simulink library "Kitchen_Lib"  (R2023a)
settings: Solver=VariableStepAuto  StartTime=0.0  StopTime=10.0  RelTol=1e-3  EnableMultiTasking=on
undefined symbols (not defined in the file): Kitc_BusTyp_P, Kitc_BusTypSkyr_C, Kitc_ColrLedColrls_C, Kitc_ColrLedGrn_C, Kitc_ColrLedRed_C, Kitc_ColrLedYlw_C, Kitc_StDgnWtrTank_C, Kitc_StElecPlugScktOffByClmp50_P, Kitc_StsDlyBlink_C, Kitc_StsErrBlink_C, Kitc_StsFctAcvn_P, Kitc_StsInfoBlink_C, Kitc_StsKitchnOffAutoIgOff_P, Kitc_StsKitchnOffBySwt_P, Kitc_StsKitchnOffDoorLockd_P, Kitc_StsKitchnOffIgOff_P, Kitc_StsKitchnOffUv_P, Kitc_StsKitchnOnBySwt_P, Kitc_StsKitchnOnNVM_P, Kitc_StsLedOff_C, Kitc_StsLedOn_C, Kitc_StsLrgCnsAcv_P, Kitc_StTrfrAnSwtInstd_P, Kitc_StTrfrSwtInstd_P, Kitc_TiKitcRefgtrOffDly_P, Kitc_ULowrThdBat_C, Kitc_UUpprThdBat_C, Kitc_ValFalse_C, Kitc_ValPwmFreq2_C, Kitc_ValPwmFreq_C, Kitc_ValTrue_C
libraries: MAN_Library x50, E2E_Lib x3
(part 4 of 13)

== system Kitchen_Lib/Kitchen/100ms/Kitchn/Subsystem1/Subsystem19/Trfr ==
  note: Kitc_StTrfrHiSide
  note: Kitc_StTrfrLoSide signal is deleted.
  "GW_StClmp50Off3Sec " : Inport
  "GW_StUvNormPrio " : Inport  Port=2
  ABat_StAddlBatInstd : Inport  Port=3
  GW_StEngRung : Inport  Port=4
  GW_StClmp15 : Inport  Port=5
  Kitc_StsKitcAcv : Inport  Port=6
  "GW_StStrtNew " : Inport  Port=7
  "Kitc_StTrfrSwt " : Inport  Port=8
  Kitc_StTrfrSwtUpprPart : Inport  Port=9
  Kitc_StTrfrSwtTopBtn : Inport  Port=10
  Kitc_StTrfrBotmBtm : Inport  Port=11
  Kitc_StTrfrWoutNewStrt : Inport  Port=12
  001_AutomaticControlKitchenRelease : Subsystem
  002_FlipFlop : Subsystem
  Constant : Constant  Value=Kitc_StTrfrSwtInstd_P
  Constant1 : Constant  Value=Kitc_StTrfrAnSwtInstd_P
  "Constant1                                                                 " : Subsystem  AncestorBlock=MAN_Library/TimeConstant  mask{hours=0, minutes=0, seconds=0, miliseconds=50}
      mask prompts: hours "Hour"
      mask DialogControl TimeConstant Prompt: Time Constant
      mask Display:
      | timeDraw = 'Time#';
      | if( hours == 0 && minutes == 0 && seconds == 0 && miliseconds == 0)
      |     timeDraw = strcat(timeDraw,'0secs'),
      | else
      |     if( hours ~= 0)
      |         timeDraw = strcat(timeDraw,num2str(hours),'hours');
      |     end
      |     if( minutes ~= 0)
      |         timeDraw = strcat(timeDraw,num2str(minutes),'min');
      |     end
      |     if( seconds ~= 0)
      |         timeDraw = strcat(timeDraw,num2str(seconds),'sec');
      |     end
      |     if( miliseconds ~= 0)
      |         timeDraw = strcat(timeDraw,num2str(miliseconds),'ms');
      |     end
      | end
      | fprintf(timeDraw);
  Constant2 : Constant  Value=Kitc_ValTrue_C
  Data Store Read : DataStoreRead  DataStoreName=Kitc_StTrfrSwtInstdNv  IndexOptions=Index vector (dialog)  Indices=1  OutputSizes=1
  Data Store Read1 : DataStoreRead  DataStoreName=Kitc_StTrfrAnSwtInstdNv  IndexOptions=Index vector (dialog)  Indices=1  OutputSizes=1
  Data Type Conversion : DataTypeConversion  OutDataTypeStr=boolean  SaturateOnIntegerOverflow=off  RndMeth=Floor
  Data Type Conversion1 : DataTypeConversion  OutDataTypeStr=boolean  SaturateOnIntegerOverflow=off  RndMeth=Floor
  Logical Operator : Logic  Operator=NOT  AllPortsSameDT=off  OutDataTypeStr=boolean
  Logical Operator1 : Logic  Operator=OR  Inputs=3  AllPortsSameDT=off  OutDataTypeStr=boolean
  Logical Operator2 : Logic  AllPortsSameDT=off  OutDataTypeStr=boolean
  Logical Operator5 : Logic  Operator=NOT  AllPortsSameDT=off  OutDataTypeStr=boolean
  Multiport Switch : MultiPortSwitch  DataPortOrder=Zero-based contiguous  Inputs=2  zeroidx=on  SaturateOnIntegerOverflow=off  InputSameDT=off
  Switch : Switch  Criteria=u2 ~= 0  SaturateOnIntegerOverflow=off  InputSameDT=off
  Switch1 : Switch  Criteria=u2 ~= 0  SaturateOnIntegerOverflow=off  InputSameDT=off
  Terminator : Terminator
  TurnOnDelay : Subsystem  AncestorBlock=MAN_Library/TurnOnDelay  mask(Turn On Delay){CycleTime=Cycle Time: 10 Ms}
      mask prompts: CycleTime "Select the Cycle Time:"
      mask help:
      | This is an EDGE DELAY where the turning-on edge is delayed. The delay period is entered at input PT. Output Q is set on TRUE after turning on input IN, only after the delay period is over. Output ET counts the time - beginning with the occurrence of the positive edge - until the value set at PT has been reached. The output ET shows the expired time since turning input IN on until the input state of IN is put through to output Q.
      |
      | IN : Timer starting bit
      | PT : Preset time of timer
      | Q  : Time up flag
      | ET : Current value of timer
      mask TypeOptions CycleTime: Cycle Time: 1 Ms | Cycle Time: 10 Ms | Cycle Time: 100 Ms | Cycle Time: 1000 Ms
      mask Display:
      | disp('{\bf\fontsize{18}Turn On Delay}', 'texmode','on');
      | 
      | port_label('input', 1,'IN');
      | port_label('input', 2,'PT');
      | port_label('output',1,'Q');
      | port_label('output',2,'ET');
  Kitc_StTrfr : Outport
  Kitc_StTrfrInstd : Outport  Port=2
  wires:
  [Kitc_StTrfrSwtUpprPart] -> Logical Operator/1
  Data Type Conversion1/1 -> Switch1/2
  Data Type Conversion/1 -> Switch/2
  Switch1/1 -> Logical Operator1/3
  Constant1/1 -> Switch1/3
  Data Store Read1/1 -> Data Type Conversion1/1, Switch1/1
  Switch/1 -> Logical Operator1/2
  Data Store Read/1 -> Data Type Conversion/1, Switch/1
  Constant/1 -> Switch/3
  Kitc_StTrfrWoutNewStrt/1 -> 002_FlipFlop/11(Kitc_StTrfrWoutNewStrt)
  "GW_StStrtNew "/1 -> 002_FlipFlop/10("GW_StStrtNew ")
  Kitc_StTrfrBotmBtm/1 -> 002_FlipFlop/9(Kitc_StTrfrBotmBtm)
  Logical Operator/1 -> 002_FlipFlop/8(Kitc_StTrfrSwtLowrPart)
  Kitc_StTrfrSwtTopBtn/1 -> 002_FlipFlop/7(Kitc_StTrfrSwtTopBtn)
  Kitc_StTrfrSwtUpprPart/1 -> [Kitc_StTrfrSwtUpprPart], 002_FlipFlop/6(Kitc_StTrfrSwtUpprPart)
  GW_StClmp15/1 -> 002_FlipFlop/1(GW_StClmp15), 001_AutomaticControlKitchenRelease/5(GW_StClmp15)
  "GW_StUvNormPrio "/1 -> 002_FlipFlop/2("GW_StUvNormPrio "), 001_AutomaticControlKitchenRelease/4("GW_StUvNormPrio ")
  Kitc_StsKitcAcv/1 -> 001_AutomaticControlKitchenRelease/1(Kitc_StsKitcAcv)
  GW_StEngRung/1 -> 002_FlipFlop/3(GW_StEngRung), 001_AutomaticControlKitchenRelease/3(GW_StEngRung)
  ABat_StAddlBatInstd/1 -> 002_FlipFlop/4(ABat_StAddlBatInstd), 001_AutomaticControlKitchenRelease/2(ABat_StAddlBatInstd)
  Logical Operator1/1 -> Multiport Switch/1, 002_FlipFlop/5(TrfrSwt)
  001_AutomaticControlKitchenRelease/1(Kitchen) -> Multiport Switch/2
  Logical Operator5/1 -> Logical Operator2/1
  Constant2/1 -> Kitc_StTrfrInstd/1
  Multiport Switch/1 -> Logical Operator2/2
  "Kitc_StTrfrSwt "/1 -> Logical Operator1/1
  "Constant1                                                                 "/1(time) -> TurnOnDelay/2(TurnOnDelayThreshold)
  TurnOnDelay/1(TurnOnDelayFlag) -> Kitc_StTrfr/1
  Logical Operator2/1 -> TurnOnDelay/1(TurnOnDelayEnable)
  "GW_StClmp50Off3Sec "/1 -> Logical Operator5/1
  TurnOnDelay/2(TurnOnDelayExpiredTime) -> Terminator/1
  002_FlipFlop/1(Fnc_On) -> Multiport Switch/3

== system Kitchen_Lib/Kitchen/100ms/Kitchn/Subsystem1/Subsystem19/WaterTankEmptyDiagnostic ==
  Kitc_StsWtrTankEmpty : Inport
  "GW_StrtLock " : Inport  Port=2
  "GW_StClmp15On3Sec " : Inport  Port=3
  "Constant                                         " : Subsystem  AncestorBlock=MAN_Library/TimeConstant  mask{hours=0, minutes=0, seconds=3, miliseconds=0}
      mask prompts: hours "Hour"
      mask DialogControl TimeConstant Prompt: Time Constant
      mask Display:
      | timeDraw = 'Time#';
      | if( hours == 0 && minutes == 0 && seconds == 0 && miliseconds == 0)
      |     timeDraw = strcat(timeDraw,'0secs'),
      | else
      |     if( hours ~= 0)
      |         timeDraw = strcat(timeDraw,num2str(hours),'hours');
      |     end
      |     if( minutes ~= 0)
      |         timeDraw = strcat(timeDraw,num2str(minutes),'min');
      |     end
      |     if( seconds ~= 0)
      |         timeDraw = strcat(timeDraw,num2str(seconds),'sec');
      |     end
      |     if( miliseconds ~= 0)
      |         timeDraw = strcat(timeDraw,num2str(miliseconds),'ms');
      |     end
      | end
      | fprintf(timeDraw);
  "Constant1                                        " : Subsystem  AncestorBlock=MAN_Library/TimeConstant  mask{hours=0, minutes=0, seconds=30, miliseconds=0}
      mask prompts: hours "Hour"
      mask DialogControl TimeConstant Prompt: Time Constant
      mask Display:
      | timeDraw = 'Time#';
      | if( hours == 0 && minutes == 0 && seconds == 0 && miliseconds == 0)
      |     timeDraw = strcat(timeDraw,'0secs'),
      | else
      |     if( hours ~= 0)
      |         timeDraw = strcat(timeDraw,num2str(hours),'hours');
      |     end
      |     if( minutes ~= 0)
      |         timeDraw = strcat(timeDraw,num2str(minutes),'min');
      |     end
      |     if( seconds ~= 0)
      |         timeDraw = strcat(timeDraw,num2str(seconds),'sec');
      |     end
      |     if( miliseconds ~= 0)
      |         timeDraw = strcat(timeDraw,num2str(miliseconds),'ms');
      |     end
      | end
      | fprintf(timeDraw);
  "Constant2                                        " : Subsystem  AncestorBlock=MAN_Library/TimeConstant  mask{hours=0, minutes=1, seconds=0, miliseconds=0}
      mask prompts: hours "Hour"
      mask DialogControl TimeConstant Prompt: Time Constant
      mask Display:
      | timeDraw = 'Time#';
      | if( hours == 0 && minutes == 0 && seconds == 0 && miliseconds == 0)
      |     timeDraw = strcat(timeDraw,'0secs'),
      | else
      |     if( hours ~= 0)
      |         timeDraw = strcat(timeDraw,num2str(hours),'hours');
      |     end
      |     if( minutes ~= 0)
      |         timeDraw = strcat(timeDraw,num2str(minutes),'min');
      |     end
      |     if( seconds ~= 0)
      |         timeDraw = strcat(timeDraw,num2str(seconds),'sec');
      |     end
      |     if( miliseconds ~= 0)
      |         timeDraw = strcat(timeDraw,num2str(miliseconds),'ms');
      |     end
      | end
      | fprintf(timeDraw);
  Constant8 : Constant  Value=Kitc_ValTrue_C
  DIAG : Subsystem
  Diagno sticsDebouncing : Subsystem  AncestorBlock=MAN_Library/DiagnosticsDebouncing  mask(Diagnostics Debouncing){CycleTime=Cycle Time: 10 Ms}
      mask prompts: CycleTime "Select the Cycle Time:"
      mask TypeOptions CycleTime: Cycle Time: 1 Ms | Cycle Time: 10 Ms | Cycle Time: 100 Ms | Cycle Time: 1000 Ms
      mask Display:
      | %fprintf('PulseGenerator');
      | 
      | port_label('input', 1,'Error');
      | port_label('input', 2,'StartLock');
      | port_label('input', 3,'IgnitionStatus');
      | port_label('input', 4,'OnDelay');
      | port_label('input', 5,'OffDelay');
      | port_label('output',1,'DiagnosticFlag');
  Terminator : Terminator
  TurnOffDelay : Subsystem  AncestorBlock=MAN_Library/TurnOffDelay  mask(Turn Off Delay){CycleTime=Cycle Time: 10 Ms}
      mask prompts: CycleTime "Select the Cycle Time:"
      mask help:
      | This is an EDGE DELAY where the turning-off edge is delayed. The delay period is entered at input PT. The output Q is reset after turning off input IN, only after the delay period is over. Output ET counts the time - beginning with the occurrence of the negative edge - until the value set at PT has been reached. The output ET shows the expired time since turning input IN off until the input state of IN is put through to output Q.
      |
      | IN : Timer starting bit
      | PT : Preset time of timer
      | Q  : Time pulse flag
      | ET : Current value of timer
      mask TypeOptions CycleTime: Cycle Time: 1 Ms | Cycle Time: 10 Ms | Cycle Time: 100 Ms | Cycle Time: 1000 Ms
      mask Display:
      | disp('{\bf\fontsize{18}Turn Off Delay}', 'texmode','on');
      | 
      | port_label('input', 1,'IN');
      | port_label('input', 2,'PT');
      | port_label('output',1,'Q');
      | port_label('output',2,'ET');
  Kitc_EidWtrTankEmpty : Outport
  Kitch_dispWtrTnkLvlWrng : Outport  Port=2
  wires:
  "GW_StrtLock "/1 -> Diagno sticsDebouncing/2(StartLock)
  "GW_StClmp15On3Sec "/1 -> Diagno sticsDebouncing/3(IgnitionStatus)
  TurnOffDelay/1(TurnOffDelayFlag) -> Diagno sticsDebouncing/1(Error), Kitch_dispWtrTnkLvlWrng/1
  "Constant                                         "/1(time) -> TurnOffDelay/2(TurnOffDelayThreshold)
  "Constant1                                        "/1(time) -> Diagno sticsDebouncing/4(OnDelay)
  "Constant2                                        "/1(time) -> Diagno sticsDebouncing/5(OffDelay)
  Kitc_StsWtrTankEmpty/1 -> TurnOffDelay/1(TurnOffDelayEnable)
  TurnOffDelay/2(TurnOffDelayExpiredTime) -> Terminator/1
  Diagno sticsDebouncing/1(DiagnosticFlag) -> Kitc_EidWtrTankEmpty/1, DIAG/1(In1)
  Constant8/1 -> DIAG/2(In2)

== system Kitchen_Lib/Kitchen/100ms/Kitchn/Subsystem1/Subsystem2/BOOLEAN_TO_UINT8_Signals ==
  BOOLEAN_TO_UINT8_SignalIn : Inport
  Constant : Constant  Value=uint8(0)
  Constant1 : Constant  Value=uint8(1)
  Constant2 : Constant  Value=uint8(2)
  Constant3 : Constant  Value=uint8(3)
  Data Type Conversion : DataTypeConversion  OutDataTypeStr=uint8  SaturateOnIntegerOverflow=off  RndMeth=Floor
  Relational Operator{,1..3} (4 alike) : RelationalOperator  Operator===  OutDataTypeStr=boolean  InputSameDT=off
  SignalOff : Outport
  Signal|On : Outport  Port=2
  Error : Outport  Port=3
  NotInstalled_NotAvailable : Outport  Port=4
  wires:
  Relational Operator3/1 -> NotInstalled_NotAvailable/1
  Relational Operator2/1 -> Error/1
  Relational Operator1/1 -> Signal|On/1
  Relational Operator/1 -> SignalOff/1
  Data Type Conversion/1 -> Relational Operator/1, Relational Operator2/1, Relational Operator3/1, Relational Operator1/1
  Constant2/1 -> Relational Operator2/2
  Constant/1 -> Relational Operator/2
  BOOLEAN_TO_UINT8_SignalIn/1 -> Data Type Conversion/1
  Constant3/1 -> Relational Operator3/2
  Constant1/1 -> Relational Operator1/2

== system Kitchen_Lib/Kitchen/100ms/Kitchn/Subsystem1/Subsystem20/UINT32_Signal ==
  UINT32_SignalIn : Inport
  Constant : Constant  Value=uint32(0)
  Constant1 : Constant  Value=uint32(1)
  Constant2 : Constant  Value=uint32(4294967294)
  Constant3 : Constant  Value=uint32(4294967295)
  Data Type Conversion : DataTypeConversion  OutDataTypeStr=uint32  SaturateOnIntegerOverflow=off  RndMeth=Floor
  Relational Operator{,1..3} (4 alike) : RelationalOperator  Operator===  OutDataTypeStr=boolean  InputSameDT=off
  Terminator : Terminator
  Terminator1 : Terminator
  Error : Outport
  NotInstalled_NotAvailable : Outport  Port=2
  wires:
  Relational Operator3/1 -> NotInstalled_NotAvailable/1
  Relational Operator2/1 -> Error/1
  Data Type Conversion/1 -> Relational Operator/1, Relational Operator1/1, Relational Operator2/1, Relational Operator3/1
  Constant/1 -> Relational Operator/2
  UINT32_SignalIn/1 -> Data Type Conversion/1
  Constant3/1 -> Relational Operator3/2
  Constant1/1 -> Relational Operator1/2
  Relational Operator/1 -> Terminator/1
  Relational Operator1/1 -> Terminator1/1
  Constant2/1 -> Relational Operator2/2

== system Kitchen_Lib/Kitchen/100ms/Kitchn/Subsystem1/Subsystem21/SignalE2EStandardBool ==
  Sıgnal_In : Inport
  Error_In : Inport  Port=2
  NotAvailable : Inport  Port=3
  Constant10 : Constant  Value=uint8(2)
  Constant12 : Constant  Value=uint8(3)
  Constant7 : Constant  Value=uint8(1)
  Constant9 : Constant  Value=uint8(0)
  Data Type Conversion1 : DataTypeConversion  OutDataTypeStr=boolean  SaturateOnIntegerOverflow=off  RndMeth=Floor
  Data Type Conversion2 : DataTypeConversion  OutDataTypeStr=boolean  SaturateOnIntegerOverflow=off  RndMeth=Floor
  Data Type Conversion3 : DataTypeConversion  OutDataTypeStr=boolean  SaturateOnIntegerOverflow=off  RndMeth=Floor
  Multiport Switch : MultiPortSwitch  DataPortOrder=Zero-based contiguous  Inputs=2  zeroidx=on  SaturateOnIntegerOverflow=off  InputSameDT=off
  Multiport Switch1 : MultiPortSwitch  DataPortOrder=Zero-based contiguous  Inputs=2  zeroidx=on  SaturateOnIntegerOverflow=off  InputSameDT=off
  Multiport Switch2 : MultiPortSwitch  DataPortOrder=Zero-based contiguous  Inputs=2  zeroidx=on  SaturateOnIntegerOverflow=off  InputSameDT=off
  Signal_Out : Outport
  wires:
  Multiport Switch2/1 -> Signal_Out/1
  Data Type Conversion3/1 -> Multiport Switch2/1
  Data Type Conversion2/1 -> Multiport Switch1/1
  Constant12/1 -> Multiport Switch2/3
  NotAvailable/1 -> Data Type Conversion3/1
  Multiport Switch1/1 -> Multiport Switch2/2
  Error_In/1 -> Data Type Conversion2/1
  Multiport Switch/1 -> Multiport Switch1/2
  Constant10/1 -> Multiport Switch1/3
  Constant9/1 -> Multiport Switch/2
  Constant7/1 -> Multiport Switch/3
  Data Type Conversion1/1 -> Multiport Switch/1
  Sıgnal_In/1 -> Data Type Conversion1/1

== system Kitchen_Lib/Kitchen/100ms/Kitchn/Subsystem1/Subsystem22/SignalE2EStandardU16 ==
  Sıgnal_In : Inport
  Error_In : Inport  Port=2
  NotAvailable : Inport  Port=3
  Constant10 : Constant  Value=uint16(65534)
  Constant12 : Constant  Value=uint16(65535)
  Constant9 : Constant  Value=uint16(0)
  Data Type Conversion1 : DataTypeConversion  OutDataTypeStr=boolean  SaturateOnIntegerOverflow=off  RndMeth=Floor
  Data Type Conversion2 : DataTypeConversion  OutDataTypeStr=boolean  SaturateOnIntegerOverflow=off  RndMeth=Floor
  Data Type Conversion3 : DataTypeConversion  OutDataTypeStr=boolean  SaturateOnIntegerOverflow=off  RndMeth=Floor
  Multiport Switch : MultiPortSwitch  DataPortOrder=Zero-based contiguous  Inputs=2  zeroidx=on  SaturateOnIntegerOverflow=off  InputSameDT=off
  Multiport Switch1 : MultiPortSwitch  DataPortOrder=Zero-based contiguous  Inputs=2  zeroidx=on  SaturateOnIntegerOverflow=off  InputSameDT=off
  Multiport Switch2 : MultiPortSwitch  DataPortOrder=Zero-based contiguous  Inputs=2  zeroidx=on  SaturateOnIntegerOverflow=off  InputSameDT=off
  Signal_Out : Outport
  wires:
  Data Type Conversion1/1 -> Multiport Switch/1
  Sıgnal_In/1 -> Data Type Conversion1/1, Multiport Switch/3
  Constant9/1 -> Multiport Switch/2
  Constant10/1 -> Multiport Switch1/3
  Multiport Switch/1 -> Multiport Switch1/2
  Error_In/1 -> Data Type Conversion2/1
  Multiport Switch1/1 -> Multiport Switch2/2
  NotAvailable/1 -> Data Type Conversion3/1
  Constant12/1 -> Multiport Switch2/3
  Data Type Conversion2/1 -> Multiport Switch1/1
  Data Type Conversion3/1 -> Multiport Switch2/1
  Multiport Switch2/1 -> Signal_Out/1

== system Kitchen_Lib/Kitchen/100ms/Kitchn/Subsystem1/Subsystem23/SignalE2EStandardU16 ==
  Sıgnal_In : Inport
  Error_In : Inport  Port=2
  NotAvailable : Inport  Port=3
  Constant10 : Constant  Value=uint16(65534)
  Constant12 : Constant  Value=uint16(65535)
  Constant9 : Constant  Value=uint16(0)
  Data Type Conversion1 : DataTypeConversion  OutDataTypeStr=boolean  SaturateOnIntegerOverflow=off  RndMeth=Floor
  Data Type Conversion2 : DataTypeConversion  OutDataTypeStr=boolean  SaturateOnIntegerOverflow=off  RndMeth=Floor
  Data Type Conversion3 : DataTypeConversion  OutDataTypeStr=boolean  SaturateOnIntegerOverflow=off  RndMeth=Floor
  Multiport Switch : MultiPortSwitch  DataPortOrder=Zero-based contiguous  Inputs=2  zeroidx=on  SaturateOnIntegerOverflow=off  InputSameDT=off
  Multiport Switch1 : MultiPortSwitch  DataPortOrder=Zero-based contiguous  Inputs=2  zeroidx=on  SaturateOnIntegerOverflow=off  InputSameDT=off
  Multiport Switch2 : MultiPortSwitch  DataPortOrder=Zero-based contiguous  Inputs=2  zeroidx=on  SaturateOnIntegerOverflow=off  InputSameDT=off
  Signal_Out : Outport
  wires:
  Data Type Conversion1/1 -> Multiport Switch/1
  Sıgnal_In/1 -> Data Type Conversion1/1, Multiport Switch/3
  Constant9/1 -> Multiport Switch/2
  Constant10/1 -> Multiport Switch1/3
  Multiport Switch/1 -> Multiport Switch1/2
  Error_In/1 -> Data Type Conversion2/1
  Multiport Switch1/1 -> Multiport Switch2/2
  NotAvailable/1 -> Data Type Conversion3/1
  Constant12/1 -> Multiport Switch2/3
  Data Type Conversion2/1 -> Multiport Switch1/1
  Data Type Conversion3/1 -> Multiport Switch2/1
  Multiport Switch2/1 -> Signal_Out/1

== system Kitchen_Lib/Kitchen/100ms/Kitchn/Subsystem1/Subsystem24/SignalE2EStandardBool ==
  Sıgnal_In : Inport
  Error_In : Inport  Port=2
  NotAvailable : Inport  Port=3
  Constant10 : Constant  Value=uint8(2)
  Constant12 : Constant  Value=uint8(3)
  Constant7 : Constant  Value=uint8(1)
  Constant9 : Constant  Value=uint8(0)
  Data Type Conversion1 : DataTypeConversion  OutDataTypeStr=boolean  SaturateOnIntegerOverflow=off  RndMeth=Floor
  Data Type Conversion2 : DataTypeConversion  OutDataTypeStr=boolean  SaturateOnIntegerOverflow=off  RndMeth=Floor
  Data Type Conversion3 : DataTypeConversion  OutDataTypeStr=boolean  SaturateOnIntegerOverflow=off  RndMeth=Floor
  Multiport Switch : MultiPortSwitch  DataPortOrder=Zero-based contiguous  Inputs=2  zeroidx=on  SaturateOnIntegerOverflow=off  InputSameDT=off
  Multiport Switch1 : MultiPortSwitch  DataPortOrder=Zero-based contiguous  Inputs=2  zeroidx=on  SaturateOnIntegerOverflow=off  InputSameDT=off
  Multiport Switch2 : MultiPortSwitch  DataPortOrder=Zero-based contiguous  Inputs=2  zeroidx=on  SaturateOnIntegerOverflow=off  InputSameDT=off
  Signal_Out : Outport
  wires:
  Multiport Switch2/1 -> Signal_Out/1
  Data Type Conversion3/1 -> Multiport Switch2/1
  Data Type Conversion2/1 -> Multiport Switch1/1
  Constant12/1 -> Multiport Switch2/3
  NotAvailable/1 -> Data Type Conversion3/1
  Multiport Switch1/1 -> Multiport Switch2/2
  Error_In/1 -> Data Type Conversion2/1
  Multiport Switch/1 -> Multiport Switch1/2
  Constant10/1 -> Multiport Switch1/3
  Constant9/1 -> Multiport Switch/2
  Constant7/1 -> Multiport Switch/3
  Data Type Conversion1/1 -> Multiport Switch/1
  Sıgnal_In/1 -> Data Type Conversion1/1

== system Kitchen_Lib/Kitchen/100ms/Kitchn/Subsystem1/Subsystem25/SignalE2EStandardBool ==
  Sıgnal_In : Inport
  Error_In : Inport  Port=2
  NotAvailable : Inport  Port=3
  Constant10 : Constant  Value=uint8(2)
  Constant12 : Constant  Value=uint8(3)
  Constant7 : Constant  Value=uint8(1)
  Constant9 : Constant  Value=uint8(0)
  Data Type Conversion1 : DataTypeConversion  OutDataTypeStr=boolean  SaturateOnIntegerOverflow=off  RndMeth=Floor
  Data Type Conversion2 : DataTypeConversion  OutDataTypeStr=boolean  SaturateOnIntegerOverflow=off  RndMeth=Floor
  Data Type Conversion3 : DataTypeConversion  OutDataTypeStr=boolean  SaturateOnIntegerOverflow=off  RndMeth=Floor
  Multiport Switch : MultiPortSwitch  DataPortOrder=Zero-based contiguous  Inputs=2  zeroidx=on  SaturateOnIntegerOverflow=off  InputSameDT=off
  Multiport Switch1 : MultiPortSwitch  DataPortOrder=Zero-based contiguous  Inputs=2  zeroidx=on  SaturateOnIntegerOverflow=off  InputSameDT=off
  Multiport Switch2 : MultiPortSwitch  DataPortOrder=Zero-based contiguous  Inputs=2  zeroidx=on  SaturateOnIntegerOverflow=off  InputSameDT=off
  Signal_Out : Outport
  wires:
  Multiport Switch2/1 -> Signal_Out/1
  Data Type Conversion3/1 -> Multiport Switch2/1
  Data Type Conversion2/1 -> Multiport Switch1/1
  Constant12/1 -> Multiport Switch2/3
  NotAvailable/1 -> Data Type Conversion3/1
  Multiport Switch1/1 -> Multiport Switch2/2
  Error_In/1 -> Data Type Conversion2/1
  Multiport Switch/1 -> Multiport Switch1/2
  Constant10/1 -> Multiport Switch1/3
  Constant9/1 -> Multiport Switch/2
  Constant7/1 -> Multiport Switch/3
  Data Type Conversion1/1 -> Multiport Switch/1
  Sıgnal_In/1 -> Data Type Conversion1/1

== system Kitchen_Lib/Kitchen/100ms/Kitchn/Subsystem1/Subsystem26/SignalE2EStandardBool ==
  Sıgnal_In : Inport
  Error_In : Inport  Port=2
  NotAvailable : Inport  Port=3
  Constant10 : Constant  Value=uint8(2)
  Constant12 : Constant  Value=uint8(3)
  Constant7 : Constant  Value=uint8(1)
  Constant9 : Constant  Value=uint8(0)
  Data Type Conversion1 : DataTypeConversion  OutDataTypeStr=boolean  SaturateOnIntegerOverflow=off  RndMeth=Floor
  Data Type Conversion2 : DataTypeConversion  OutDataTypeStr=boolean  SaturateOnIntegerOverflow=off  RndMeth=Floor
  Data Type Conversion3 : DataTypeConversion  OutDataTypeStr=boolean  SaturateOnIntegerOverflow=off  RndMeth=Floor
  Multiport Switch : MultiPortSwitch  DataPortOrder=Zero-based contiguous  Inputs=2  zeroidx=on  SaturateOnIntegerOverflow=off  InputSameDT=off
  Multiport Switch1 : MultiPortSwitch  DataPortOrder=Zero-based contiguous  Inputs=2  zeroidx=on  SaturateOnIntegerOverflow=off  InputSameDT=off
  Multiport Switch2 : MultiPortSwitch  DataPortOrder=Zero-based contiguous  Inputs=2  zeroidx=on  SaturateOnIntegerOverflow=off  InputSameDT=off
  Signal_Out : Outport
  wires:
  Multiport Switch2/1 -> Signal_Out/1
  Data Type Conversion3/1 -> Multiport Switch2/1
  Data Type Conversion2/1 -> Multiport Switch1/1
  Constant12/1 -> Multiport Switch2/3
  NotAvailable/1 -> Data Type Conversion3/1
  Multiport Switch1/1 -> Multiport Switch2/2
  Error_In/1 -> Data Type Conversion2/1
  Multiport Switch/1 -> Multiport Switch1/2
  Constant10/1 -> Multiport Switch1/3
  Constant9/1 -> Multiport Switch/2
  Constant7/1 -> Multiport Switch/3
  Data Type Conversion1/1 -> Multiport Switch/1
  Sıgnal_In/1 -> Data Type Conversion1/1

== system Kitchen_Lib/Kitchen/100ms/Kitchn/Subsystem1/Subsystem27/SignalE2EStandardBool ==
  Sıgnal_In : Inport
  Error_In : Inport  Port=2
  NotAvailable : Inport  Port=3
  Constant10 : Constant  Value=uint8(2)
  Constant12 : Constant  Value=uint8(3)
  Constant7 : Constant  Value=uint8(1)
  Constant9 : Constant  Value=uint8(0)
  Data Type Conversion1 : DataTypeConversion  OutDataTypeStr=boolean  SaturateOnIntegerOverflow=off  RndMeth=Floor
  Data Type Conversion2 : DataTypeConversion  OutDataTypeStr=boolean  SaturateOnIntegerOverflow=off  RndMeth=Floor
  Data Type Conversion3 : DataTypeConversion  OutDataTypeStr=boolean  SaturateOnIntegerOverflow=off  RndMeth=Floor
  Multiport Switch : MultiPortSwitch  DataPortOrder=Zero-based contiguous  Inputs=2  zeroidx=on  SaturateOnIntegerOverflow=off  InputSameDT=off
  Multiport Switch1 : MultiPortSwitch  DataPortOrder=Zero-based contiguous  Inputs=2  zeroidx=on  SaturateOnIntegerOverflow=off  InputSameDT=off
  Multiport Switch2 : MultiPortSwitch  DataPortOrder=Zero-based contiguous  Inputs=2  zeroidx=on  SaturateOnIntegerOverflow=off  InputSameDT=off
  Signal_Out : Outport
  wires:
  Multiport Switch2/1 -> Signal_Out/1
  Data Type Conversion3/1 -> Multiport Switch2/1
  Data Type Conversion2/1 -> Multiport Switch1/1
  Constant12/1 -> Multiport Switch2/3
  NotAvailable/1 -> Data Type Conversion3/1
  Multiport Switch1/1 -> Multiport Switch2/2
  Error_In/1 -> Data Type Conversion2/1
  Multiport Switch/1 -> Multiport Switch1/2
  Constant10/1 -> Multiport Switch1/3
  Constant9/1 -> Multiport Switch/2
  Constant7/1 -> Multiport Switch/3
  Data Type Conversion1/1 -> Multiport Switch/1
  Sıgnal_In/1 -> Data Type Conversion1/1

== system Kitchen_Lib/Kitchen/100ms/Kitchn/Subsystem1/Subsystem28/SignalE2EStandardBool ==
  Sıgnal_In : Inport
  Error_In : Inport  Port=2
  NotAvailable : Inport  Port=3
  Constant10 : Constant  Value=uint8(2)
  Constant12 : Constant  Value=uint8(3)
  Constant7 : Constant  Value=uint8(1)
  Constant9 : Constant  Value=uint8(0)
  Data Type Conversion1 : DataTypeConversion  OutDataTypeStr=boolean  SaturateOnIntegerOverflow=off  RndMeth=Floor
  Data Type Conversion2 : DataTypeConversion  OutDataTypeStr=boolean  SaturateOnIntegerOverflow=off  RndMeth=Floor
  Data Type Conversion3 : DataTypeConversion  OutDataTypeStr=boolean  SaturateOnIntegerOverflow=off  RndMeth=Floor
  Multiport Switch : MultiPortSwitch  DataPortOrder=Zero-based contiguous  Inputs=2  zeroidx=on  SaturateOnIntegerOverflow=off  InputSameDT=off
  Multiport Switch1 : MultiPortSwitch  DataPortOrder=Zero-based contiguous  Inputs=2  zeroidx=on  SaturateOnIntegerOverflow=off  InputSameDT=off
  Multiport Switch2 : MultiPortSwitch  DataPortOrder=Zero-based contiguous  Inputs=2  zeroidx=on  SaturateOnIntegerOverflow=off  InputSameDT=off
  Signal_Out : Outport
  wires:
  Multiport Switch2/1 -> Signal_Out/1
  Data Type Conversion3/1 -> Multiport Switch2/1
  Data Type Conversion2/1 -> Multiport Switch1/1
  Constant12/1 -> Multiport Switch2/3
  NotAvailable/1 -> Data Type Conversion3/1
  Multiport Switch1/1 -> Multiport Switch2/2
  Error_In/1 -> Data Type Conversion2/1
  Multiport Switch/1 -> Multiport Switch1/2
  Constant10/1 -> Multiport Switch1/3
  Constant9/1 -> Multiport Switch/2
  Constant7/1 -> Multiport Switch/3
  Data Type Conversion1/1 -> Multiport Switch/1
  Sıgnal_In/1 -> Data Type Conversion1/1

== system Kitchen_Lib/Kitchen/100ms/Kitchn/Subsystem1/Subsystem29/SignalE2EStandardBool ==
  Sıgnal_In : Inport
  Error_In : Inport  Port=2
  NotAvailable : Inport  Port=3
  Constant10 : Constant  Value=uint8(2)
  Constant12 : Constant  Value=uint8(3)
  Constant7 : Constant  Value=uint8(1)
  Constant9 : Constant  Value=uint8(0)
  Data Type Conversion1 : DataTypeConversion  OutDataTypeStr=boolean  SaturateOnIntegerOverflow=off  RndMeth=Floor
  Data Type Conversion2 : DataTypeConversion  OutDataTypeStr=boolean  SaturateOnIntegerOverflow=off  RndMeth=Floor
  Data Type Conversion3 : DataTypeConversion  OutDataTypeStr=boolean  SaturateOnIntegerOverflow=off  RndMeth=Floor
  Multiport Switch : MultiPortSwitch  DataPortOrder=Zero-based contiguous  Inputs=2  zeroidx=on  SaturateOnIntegerOverflow=off  InputSameDT=off
  Multiport Switch1 : MultiPortSwitch  DataPortOrder=Zero-based contiguous  Inputs=2  zeroidx=on  SaturateOnIntegerOverflow=off  InputSameDT=off
  Multiport Switch2 : MultiPortSwitch  DataPortOrder=Zero-based contiguous  Inputs=2  zeroidx=on  SaturateOnIntegerOverflow=off  InputSameDT=off
  Signal_Out : Outport
  wires:
  Multiport Switch2/1 -> Signal_Out/1
  Data Type Conversion3/1 -> Multiport Switch2/1
  Data Type Conversion2/1 -> Multiport Switch1/1
  Constant12/1 -> Multiport Switch2/3
  NotAvailable/1 -> Data Type Conversion3/1
  Multiport Switch1/1 -> Multiport Switch2/2
  Error_In/1 -> Data Type Conversion2/1
  Multiport Switch/1 -> Multiport Switch1/2
  Constant10/1 -> Multiport Switch1/3
  Constant9/1 -> Multiport Switch/2
  Constant7/1 -> Multiport Switch/3
  Data Type Conversion1/1 -> Multiport Switch/1
  Sıgnal_In/1 -> Data Type Conversion1/1

== system Kitchen_Lib/Kitchen/100ms/Kitchn/Subsystem1/Subsystem3/BOOLEAN_TO_UINT8_Signals ==
  BOOLEAN_TO_UINT8_SignalIn : Inport
  Constant : Constant  Value=uint8(0)
  Constant1 : Constant  Value=uint8(1)
  Constant2 : Constant  Value=uint8(2)
  Constant3 : Constant  Value=uint8(3)
  Data Type Conversion : DataTypeConversion  OutDataTypeStr=uint8  SaturateOnIntegerOverflow=off  RndMeth=Floor
  Relational Operator{,1..3} (4 alike) : RelationalOperator  Operator===  OutDataTypeStr=boolean  InputSameDT=off
  SignalOff : Outport
  Signal|On : Outport  Port=2
  Error : Outport  Port=3
  NotInstalled_NotAvailable : Outport  Port=4
  wires:
  Relational Operator3/1 -> NotInstalled_NotAvailable/1
  Relational Operator2/1 -> Error/1
  Relational Operator1/1 -> Signal|On/1
  Relational Operator/1 -> SignalOff/1
  Data Type Conversion/1 -> Relational Operator/1, Relational Operator2/1, Relational Operator3/1, Relational Operator1/1
  Constant2/1 -> Relational Operator2/2
  Constant/1 -> Relational Operator/2
  BOOLEAN_TO_UINT8_SignalIn/1 -> Data Type Conversion/1
  Constant3/1 -> Relational Operator3/2
  Constant1/1 -> Relational Operator1/2

== system Kitchen_Lib/Kitchen/100ms/Kitchn/Subsystem1/Subsystem30/SignalE2EStandardBool ==
  Sıgnal_In : Inport
  Error_In : Inport  Port=2
  NotAvailable : Inport  Port=3
  Constant10 : Constant  Value=uint8(2)
  Constant12 : Constant  Value=uint8(3)
  Constant7 : Constant  Value=uint8(1)
  Constant9 : Constant  Value=uint8(0)
  Data Type Conversion1 : DataTypeConversion  OutDataTypeStr=boolean  SaturateOnIntegerOverflow=off  RndMeth=Floor
  Data Type Conversion2 : DataTypeConversion  OutDataTypeStr=boolean  SaturateOnIntegerOverflow=off  RndMeth=Floor
  Data Type Conversion3 : DataTypeConversion  OutDataTypeStr=boolean  SaturateOnIntegerOverflow=off  RndMeth=Floor
  Multiport Switch : MultiPortSwitch  DataPortOrder=Zero-based contiguous  Inputs=2  zeroidx=on  SaturateOnIntegerOverflow=off  InputSameDT=off
  Multiport Switch1 : MultiPortSwitch  DataPortOrder=Zero-based contiguous  Inputs=2  zeroidx=on  SaturateOnIntegerOverflow=off  InputSameDT=off
  Multiport Switch2 : MultiPortSwitch  DataPortOrder=Zero-based contiguous  Inputs=2  zeroidx=on  SaturateOnIntegerOverflow=off  InputSameDT=off
  Signal_Out : Outport
  wires:
  Multiport Switch2/1 -> Signal_Out/1
  Data Type Conversion3/1 -> Multiport Switch2/1
  Data Type Conversion2/1 -> Multiport Switch1/1
  Constant12/1 -> Multiport Switch2/3
  NotAvailable/1 -> Data Type Conversion3/1
  Multiport Switch1/1 -> Multiport Switch2/2
  Error_In/1 -> Data Type Conversion2/1
  Multiport Switch/1 -> Multiport Switch1/2
  Constant10/1 -> Multiport Switch1/3
  Constant9/1 -> Multiport Switch/2
  Constant7/1 -> Multiport Switch/3
  Data Type Conversion1/1 -> Multiport Switch/1
  Sıgnal_In/1 -> Data Type Conversion1/1

== system Kitchen_Lib/Kitchen/100ms/Kitchn/Subsystem1/Subsystem31/SignalE2EStandardBool ==
  Sıgnal_In : Inport
  Error_In : Inport  Port=2
  NotAvailable : Inport  Port=3
  Constant10 : Constant  Value=uint8(2)
  Constant12 : Constant  Value=uint8(3)
  Constant7 : Constant  Value=uint8(1)
  Constant9 : Constant  Value=uint8(0)
  Data Type Conversion1 : DataTypeConversion  OutDataTypeStr=boolean  SaturateOnIntegerOverflow=off  RndMeth=Floor
  Data Type Conversion2 : DataTypeConversion  OutDataTypeStr=boolean  SaturateOnIntegerOverflow=off  RndMeth=Floor
  Data Type Conversion3 : DataTypeConversion  OutDataTypeStr=boolean  SaturateOnIntegerOverflow=off  RndMeth=Floor
  Multiport Switch : MultiPortSwitch  DataPortOrder=Zero-based contiguous  Inputs=2  zeroidx=on  SaturateOnIntegerOverflow=off  InputSameDT=off
  Multiport Switch1 : MultiPortSwitch  DataPortOrder=Zero-based contiguous  Inputs=2  zeroidx=on  SaturateOnIntegerOverflow=off  InputSameDT=off
  Multiport Switch2 : MultiPortSwitch  DataPortOrder=Zero-based contiguous  Inputs=2  zeroidx=on  SaturateOnIntegerOverflow=off  InputSameDT=off
  Signal_Out : Outport
  wires:
  Multiport Switch2/1 -> Signal_Out/1
  Data Type Conversion3/1 -> Multiport Switch2/1
  Data Type Conversion2/1 -> Multiport Switch1/1
  Constant12/1 -> Multiport Switch2/3
  NotAvailable/1 -> Data Type Conversion3/1
  Multiport Switch1/1 -> Multiport Switch2/2
  Error_In/1 -> Data Type Conversion2/1
  Multiport Switch/1 -> Multiport Switch1/2
  Constant10/1 -> Multiport Switch1/3
  Constant9/1 -> Multiport Switch/2
  Constant7/1 -> Multiport Switch/3
  Data Type Conversion1/1 -> Multiport Switch/1
  Sıgnal_In/1 -> Data Type Conversion1/1

== system Kitchen_Lib/Kitchen/100ms/Kitchn/Subsystem1/Subsystem32/SignalE2EStandardBool ==
  Sıgnal_In : Inport
  Error_In : Inport  Port=2
  NotAvailable : Inport  Port=3
  Constant10 : Constant  Value=uint8(2)
  Constant12 : Constant  Value=uint8(3)
  Constant7 : Constant  Value=uint8(1)
  Constant9 : Constant  Value=uint8(0)
  Data Type Conversion1 : DataTypeConversion  OutDataTypeStr=boolean  SaturateOnIntegerOverflow=off  RndMeth=Floor
  Data Type Conversion2 : DataTypeConversion  OutDataTypeStr=boolean  SaturateOnIntegerOverflow=off  RndMeth=Floor
  Data Type Conversion3 : DataTypeConversion  OutDataTypeStr=boolean  SaturateOnIntegerOverflow=off  RndMeth=Floor
  Multiport Switch : MultiPortSwitch  DataPortOrder=Zero-based contiguous  Inputs=2  zeroidx=on  SaturateOnIntegerOverflow=off  InputSameDT=off
  Multiport Switch1 : MultiPortSwitch  DataPortOrder=Zero-based contiguous  Inputs=2  zeroidx=on  SaturateOnIntegerOverflow=off  InputSameDT=off
  Multiport Switch2 : MultiPortSwitch  DataPortOrder=Zero-based contiguous  Inputs=2  zeroidx=on  SaturateOnIntegerOverflow=off  InputSameDT=off
  Signal_Out : Outport
  wires:
  Multiport Switch2/1 -> Signal_Out/1
  Data Type Conversion3/1 -> Multiport Switch2/1
  Data Type Conversion2/1 -> Multiport Switch1/1
  Constant12/1 -> Multiport Switch2/3
  NotAvailable/1 -> Data Type Conversion3/1
  Multiport Switch1/1 -> Multiport Switch2/2
  Error_In/1 -> Data Type Conversion2/1
  Multiport Switch/1 -> Multiport Switch1/2
  Constant10/1 -> Multiport Switch1/3
  Constant9/1 -> Multiport Switch/2
  Constant7/1 -> Multiport Switch/3
  Data Type Conversion1/1 -> Multiport Switch/1
  Sıgnal_In/1 -> Data Type Conversion1/1

== system Kitchen_Lib/Kitchen/100ms/Kitchn/Subsystem1/Subsystem33/SignalE2EStandardU16 ==
  Sıgnal_In : Inport
  Error_In : Inport  Port=2
  NotAvailable : Inport  Port=3
  Constant10 : Constant  Value=uint16(65534)
  Constant12 : Constant  Value=uint16(65535)
  Constant9 : Constant  Value=uint16(0)
  Data Type Conversion1 : DataTypeConversion  OutDataTypeStr=boolean  SaturateOnIntegerOverflow=off  RndMeth=Floor
  Data Type Conversion2 : DataTypeConversion  OutDataTypeStr=boolean  SaturateOnIntegerOverflow=off  RndMeth=Floor
  Data Type Conversion3 : DataTypeConversion  OutDataTypeStr=boolean  SaturateOnIntegerOverflow=off  RndMeth=Floor
  Multiport Switch : MultiPortSwitch  DataPortOrder=Zero-based contiguous  Inputs=2  zeroidx=on  SaturateOnIntegerOverflow=off  InputSameDT=off
  Multiport Switch1 : MultiPortSwitch  DataPortOrder=Zero-based contiguous  Inputs=2  zeroidx=on  SaturateOnIntegerOverflow=off  InputSameDT=off
  Multiport Switch2 : MultiPortSwitch  DataPortOrder=Zero-based contiguous  Inputs=2  zeroidx=on  SaturateOnIntegerOverflow=off  InputSameDT=off
  Signal_Out : Outport
  wires:
  Data Type Conversion1/1 -> Multiport Switch/1
  Sıgnal_In/1 -> Data Type Conversion1/1, Multiport Switch/3
  Constant9/1 -> Multiport Switch/2
  Constant10/1 -> Multiport Switch1/3
  Multiport Switch/1 -> Multiport Switch1/2
  Error_In/1 -> Data Type Conversion2/1
  Multiport Switch1/1 -> Multiport Switch2/2
  NotAvailable/1 -> Data Type Conversion3/1
  Constant12/1 -> Multiport Switch2/3
  Data Type Conversion2/1 -> Multiport Switch1/1
  Data Type Conversion3/1 -> Multiport Switch2/1
  Multiport Switch2/1 -> Signal_Out/1

== system Kitchen_Lib/Kitchen/100ms/Kitchn/Subsystem1/Subsystem34/SignalE2EStandardU16 ==
  Sıgnal_In : Inport
  Error_In : Inport  Port=2
  NotAvailable : Inport  Port=3
  Constant10 : Constant  Value=uint16(65534)
  Constant12 : Constant  Value=uint16(65535)
  Constant9 : Constant  Value=uint16(0)
  Data Type Conversion1 : DataTypeConversion  OutDataTypeStr=boolean  SaturateOnIntegerOverflow=off  RndMeth=Floor
  Data Type Conversion2 : DataTypeConversion  OutDataTypeStr=boolean  SaturateOnIntegerOverflow=off  RndMeth=Floor
  Data Type Conversion3 : DataTypeConversion  OutDataTypeStr=boolean  SaturateOnIntegerOverflow=off  RndMeth=Floor
  Multiport Switch : MultiPortSwitch  DataPortOrder=Zero-based contiguous  Inputs=2  zeroidx=on  SaturateOnIntegerOverflow=off  InputSameDT=off
  Multiport Switch1 : MultiPortSwitch  DataPortOrder=Zero-based contiguous  Inputs=2  zeroidx=on  SaturateOnIntegerOverflow=off  InputSameDT=off
  Multiport Switch2 : MultiPortSwitch  DataPortOrder=Zero-based contiguous  Inputs=2  zeroidx=on  SaturateOnIntegerOverflow=off  InputSameDT=off
  Signal_Out : Outport
  wires:
  Data Type Conversion1/1 -> Multiport Switch/1
  Sıgnal_In/1 -> Data Type Conversion1/1, Multiport Switch/3
  Constant9/1 -> Multiport Switch/2
  Constant10/1 -> Multiport Switch1/3
  Multiport Switch/1 -> Multiport Switch1/2
  Error_In/1 -> Data Type Conversion2/1
  Multiport Switch1/1 -> Multiport Switch2/2
  NotAvailable/1 -> Data Type Conversion3/1
  Constant12/1 -> Multiport Switch2/3
  Data Type Conversion2/1 -> Multiport Switch1/1
  Data Type Conversion3/1 -> Multiport Switch2/1
  Multiport Switch2/1 -> Signal_Out/1

== system Kitchen_Lib/Kitchen/100ms/Kitchn/Subsystem1/Subsystem35/SignalE2EStandardU16 ==
  Sıgnal_In : Inport
  Error_In : Inport  Port=2
  NotAvailable : Inport  Port=3
  Constant10 : Constant  Value=uint16(65534)
  Constant12 : Constant  Value=uint16(65535)
  Constant9 : Constant  Value=uint16(0)
  Data Type Conversion1 : DataTypeConversion  OutDataTypeStr=boolean  SaturateOnIntegerOverflow=off  RndMeth=Floor
  Data Type Conversion2 : DataTypeConversion  OutDataTypeStr=boolean  SaturateOnIntegerOverflow=off  RndMeth=Floor
  Data Type Conversion3 : DataTypeConversion  OutDataTypeStr=boolean  SaturateOnIntegerOverflow=off  RndMeth=Floor
  Multiport Switch : MultiPortSwitch  DataPortOrder=Zero-based contiguous  Inputs=2  zeroidx=on  SaturateOnIntegerOverflow=off  InputSameDT=off
  Multiport Switch1 : MultiPortSwitch  DataPortOrder=Zero-based contiguous  Inputs=2  zeroidx=on  SaturateOnIntegerOverflow=off  InputSameDT=off
  Multiport Switch2 : MultiPortSwitch  DataPortOrder=Zero-based contiguous  Inputs=2  zeroidx=on  SaturateOnIntegerOverflow=off  InputSameDT=off
  Signal_Out : Outport
  wires:
  Data Type Conversion1/1 -> Multiport Switch/1
  Sıgnal_In/1 -> Data Type Conversion1/1, Multiport Switch/3
  Constant9/1 -> Multiport Switch/2
  Constant10/1 -> Multiport Switch1/3
  Multiport Switch/1 -> Multiport Switch1/2
  Error_In/1 -> Data Type Conversion2/1
  Multiport Switch1/1 -> Multiport Switch2/2
  NotAvailable/1 -> Data Type Conversion3/1
  Constant12/1 -> Multiport Switch2/3
  Data Type Conversion2/1 -> Multiport Switch1/1
  Data Type Conversion3/1 -> Multiport Switch2/1
  Multiport Switch2/1 -> Signal_Out/1

== system Kitchen_Lib/Kitchen/100ms/Kitchn/Subsystem1/Subsystem36/BOOLEAN_TO_UINT8_Signals ==
  BOOLEAN_TO_UINT8_SignalIn : Inport
  Constant : Constant  Value=uint8(0)
  Constant1 : Constant  Value=uint8(1)
  Constant2 : Constant  Value=uint8(2)
  Constant3 : Constant  Value=uint8(3)
  Data Type Conversion : DataTypeConversion  OutDataTypeStr=uint8  SaturateOnIntegerOverflow=off  RndMeth=Floor
  Relational Operator{,1..3} (4 alike) : RelationalOperator  Operator===  OutDataTypeStr=boolean  InputSameDT=off
  SignalOff : Outport
  Signal|On : Outport  Port=2
  Error : Outport  Port=3
  NotInstalled_NotAvailable : Outport  Port=4
  wires:
  Relational Operator3/1 -> NotInstalled_NotAvailable/1
  Relational Operator2/1 -> Error/1
  Relational Operator1/1 -> Signal|On/1
  Relational Operator/1 -> SignalOff/1
  Data Type Conversion/1 -> Relational Operator/1, Relational Operator2/1, Relational Operator3/1, Relational Operator1/1
  Constant2/1 -> Relational Operator2/2
  Constant/1 -> Relational Operator/2
  BOOLEAN_TO_UINT8_SignalIn/1 -> Data Type Conversion/1
  Constant3/1 -> Relational Operator3/2
  Constant1/1 -> Relational Operator1/2

== system Kitchen_Lib/Kitchen/100ms/Kitchn/Subsystem1/Subsystem4/BOOLEAN_TO_UINT8_Signals ==
  BOOLEAN_TO_UINT8_SignalIn : Inport
  Constant : Constant  Value=uint8(0)
  Constant1 : Constant  Value=uint8(1)
  Constant2 : Constant  Value=uint8(2)
  Constant3 : Constant  Value=uint8(3)
  Data Type Conversion : DataTypeConversion  OutDataTypeStr=uint8  SaturateOnIntegerOverflow=off  RndMeth=Floor
  Relational Operator{,1..3} (4 alike) : RelationalOperator  Operator===  OutDataTypeStr=boolean  InputSameDT=off
  SignalOff : Outport
  Signal|On : Outport  Port=2
  Error : Outport  Port=3
  NotInstalled_NotAvailable : Outport  Port=4
  wires:
  Relational Operator3/1 -> NotInstalled_NotAvailable/1
  Relational Operator2/1 -> Error/1
  Relational Operator1/1 -> Signal|On/1
  Relational Operator/1 -> SignalOff/1
  Data Type Conversion/1 -> Relational Operator/1, Relational Operator2/1, Relational Operator3/1, Relational Operator1/1
  Constant2/1 -> Relational Operator2/2
  Constant/1 -> Relational Operator/2
  BOOLEAN_TO_UINT8_SignalIn/1 -> Data Type Conversion/1
  Constant3/1 -> Relational Operator3/2
  Constant1/1 -> Relational Operator1/2

== system Kitchen_Lib/Kitchen/100ms/Kitchn/Subsystem1/Subsystem41/SignalE2EStandardU16 ==
  Sıgnal_In : Inport
  Error_In : Inport  Port=2
  NotAvailable : Inport  Port=3
  Constant10 : Constant  Value=uint16(65534)
  Constant12 : Constant  Value=uint16(65535)
  Constant9 : Constant  Value=uint16(0)
  Data Type Conversion1 : DataTypeConversion  OutDataTypeStr=boolean  SaturateOnIntegerOverflow=off  RndMeth=Floor
  Data Type Conversion2 : DataTypeConversion  OutDataTypeStr=boolean  SaturateOnIntegerOverflow=off  RndMeth=Floor
  Data Type Conversion3 : DataTypeConversion  OutDataTypeStr=boolean  SaturateOnIntegerOverflow=off  RndMeth=Floor
  Multiport Switch : MultiPortSwitch  DataPortOrder=Zero-based contiguous  Inputs=2  zeroidx=on  SaturateOnIntegerOverflow=off  InputSameDT=off
  Multiport Switch1 : MultiPortSwitch  DataPortOrder=Zero-based contiguous  Inputs=2  zeroidx=on  SaturateOnIntegerOverflow=off  InputSameDT=off
  Multiport Switch2 : MultiPortSwitch  DataPortOrder=Zero-based contiguous  Inputs=2  zeroidx=on  SaturateOnIntegerOverflow=off  InputSameDT=off
  Signal_Out : Outport
  wires:
  Data Type Conversion1/1 -> Multiport Switch/1
  Sıgnal_In/1 -> Data Type Conversion1/1, Multiport Switch/3
  Constant9/1 -> Multiport Switch/2
  Constant10/1 -> Multiport Switch1/3
  Multiport Switch/1 -> Multiport Switch1/2
  Error_In/1 -> Data Type Conversion2/1
  Multiport Switch1/1 -> Multiport Switch2/2
  NotAvailable/1 -> Data Type Conversion3/1
  Constant12/1 -> Multiport Switch2/3
  Data Type Conversion2/1 -> Multiport Switch1/1
  Data Type Conversion3/1 -> Multiport Switch2/1
  Multiport Switch2/1 -> Signal_Out/1

== system Kitchen_Lib/Kitchen/100ms/Kitchn/Subsystem1/Subsystem5/BOOLEAN_TO_UINT8_Signals ==
  BOOLEAN_TO_UINT8_SignalIn : Inport
  Constant : Constant  Value=uint8(0)
  Constant1 : Constant  Value=uint8(1)
  Constant2 : Constant  Value=uint8(2)
  Constant3 : Constant  Value=uint8(3)
  Data Type Conversion : DataTypeConversion  OutDataTypeStr=uint8  SaturateOnIntegerOverflow=off  RndMeth=Floor
  Relational Operator{,1..3} (4 alike) : RelationalOperator  Operator===  OutDataTypeStr=boolean  InputSameDT=off
  SignalOff : Outport
  Signal|On : Outport  Port=2
  Error : Outport  Port=3
  NotInstalled_NotAvailable : Outport  Port=4
  wires:
  Relational Operator3/1 -> NotInstalled_NotAvailable/1
  Relational Operator2/1 -> Error/1
  Relational Operator1/1 -> Signal|On/1
  Relational Operator/1 -> SignalOff/1
  Data Type Conversion/1 -> Relational Operator/1, Relational Operator2/1, Relational Operator3/1, Relational Operator1/1
  Constant2/1 -> Relational Operator2/2
  Constant/1 -> Relational Operator/2
  BOOLEAN_TO_UINT8_SignalIn/1 -> Data Type Conversion/1
  Constant3/1 -> Relational Operator3/2
  Constant1/1 -> Relational Operator1/2

== system Kitchen_Lib/Kitchen/100ms/Kitchn/Subsystem1/Subsystem6/BOOLEAN_TO_UINT8_Signals ==
  BOOLEAN_TO_UINT8_SignalIn : Inport
  Constant : Constant  Value=uint8(0)
  Constant1 : Constant  Value=uint8(1)
  Constant2 : Constant  Value=uint8(2)
  Constant3 : Constant  Value=uint8(3)
  Data Type Conversion : DataTypeConversion  OutDataTypeStr=uint8  SaturateOnIntegerOverflow=off  RndMeth=Floor
  Relational Operator{,1..3} (4 alike) : RelationalOperator  Operator===  OutDataTypeStr=boolean  InputSameDT=off
  SignalOff : Outport
  Signal|On : Outport  Port=2
  Error : Outport  Port=3
  NotInstalled_NotAvailable : Outport  Port=4
  wires:
  Relational Operator3/1 -> NotInstalled_NotAvailable/1
  Relational Operator2/1 -> Error/1
  Relational Operator1/1 -> Signal|On/1
  Relational Operator/1 -> SignalOff/1
  Data Type Conversion/1 -> Relational Operator/1, Relational Operator2/1, Relational Operator3/1, Relational Operator1/1
  Constant2/1 -> Relational Operator2/2
  Constant/1 -> Relational Operator/2
  BOOLEAN_TO_UINT8_SignalIn/1 -> Data Type Conversion/1
  Constant3/1 -> Relational Operator3/2
  Constant1/1 -> Relational Operator1/2

== system Kitchen_Lib/Kitchen/100ms/Kitchn/Subsystem1/Subsystem7/BOOLEAN_TO_UINT8_Signals ==
  BOOLEAN_TO_UINT8_SignalIn : Inport
  Constant : Constant  Value=uint8(0)
  Constant1 : Constant  Value=uint8(1)
  Constant2 : Constant  Value=uint8(2)
  Constant3 : Constant  Value=uint8(3)
  Data Type Conversion : DataTypeConversion  OutDataTypeStr=uint8  SaturateOnIntegerOverflow=off  RndMeth=Floor
  Relational Operator{,1..3} (4 alike) : RelationalOperator  Operator===  OutDataTypeStr=boolean  InputSameDT=off
  SignalOff : Outport
  Signal|On : Outport  Port=2
  Error : Outport  Port=3
  NotInstalled_NotAvailable : Outport  Port=4
  wires:
  Relational Operator3/1 -> NotInstalled_NotAvailable/1
  Relational Operator2/1 -> Error/1
  Relational Operator1/1 -> Signal|On/1
  Relational Operator/1 -> SignalOff/1
  Data Type Conversion/1 -> Relational Operator/1, Relational Operator2/1, Relational Operator3/1, Relational Operator1/1
  Constant2/1 -> Relational Operator2/2
  Constant/1 -> Relational Operator/2
  BOOLEAN_TO_UINT8_SignalIn/1 -> Data Type Conversion/1
  Constant3/1 -> Relational Operator3/2
  Constant1/1 -> Relational Operator1/2

== system Kitchen_Lib/Kitchen/100ms/Kitchn/Subsystem1/Subsystem8/BOOLEAN_TO_UINT8_Signals ==
  BOOLEAN_TO_UINT8_SignalIn : Inport
  Constant : Constant  Value=uint8(0)
  Constant1 : Constant  Value=uint8(1)
  Constant2 : Constant  Value=uint8(2)
  Constant3 : Constant  Value=uint8(3)
  Data Type Conversion : DataTypeConversion  OutDataTypeStr=uint8  SaturateOnIntegerOverflow=off  RndMeth=Floor
  Relational Operator{,1..3} (4 alike) : RelationalOperator  Operator===  OutDataTypeStr=boolean  InputSameDT=off
  SignalOff : Outport
  Signal|On : Outport  Port=2
  Error : Outport  Port=3
  NotInstalled_NotAvailable : Outport  Port=4
  wires:
  Relational Operator3/1 -> NotInstalled_NotAvailable/1
  Relational Operator2/1 -> Error/1
  Relational Operator1/1 -> Signal|On/1
  Relational Operator/1 -> SignalOff/1
  Data Type Conversion/1 -> Relational Operator/1, Relational Operator2/1, Relational Operator3/1, Relational Operator1/1
  Constant2/1 -> Relational Operator2/2
  Constant/1 -> Relational Operator/2
  BOOLEAN_TO_UINT8_SignalIn/1 -> Data Type Conversion/1
  Constant3/1 -> Relational Operator3/2
  Constant1/1 -> Relational Operator1/2
